simulink model "FallingBall"  (R2015b)
settings: Solver=ode1  StartTime=0.0  StopTime=10.0  FixedStep=0.02  RelTol=1e-3
model workspace (MAT data in the model file):
  g = 9.81
  m = 0.2
settings Model: Creator=andrea.emili  LastModifiedBy=andrea.emili

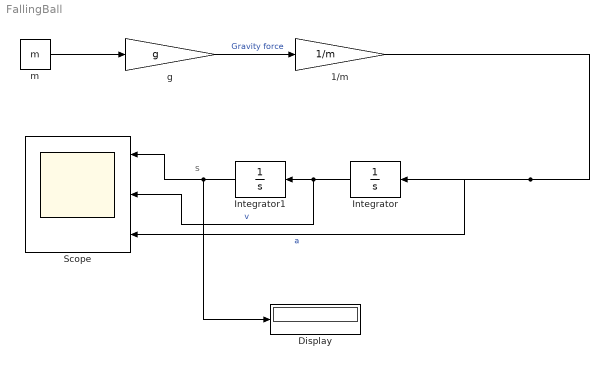
== system FallingBall ==
  note: s
  1/m : Gain  Gain=1/m
  Display : Display
  Integrator : Integrator
      settings: AttributesFormatString=S0 = %<InitialCondition>
  Integrator1 : Integrator
  Scope : Scope  NumInputPorts=3
  g : Gain  Gain=g
  m : Constant  Value=m
  wires:
  m/1 -> g/1
  g/1 -> 1/m/1  "Gravity force"
  1/m/1 -> Scope/3, Integrator/1  "a"
  Integrator/1 -> Scope/2, Integrator1/1  "v"
  Integrator1/1 -> Display/1, Scope/1
